simulink model "CAVE_MachE_Simulink_250904"  (R2024a)
settings: configuration reference "ConfigSetDesktopFixedStep" (kept outside this file)
PreLoadFcn:
  | VSS_BICYCLE=Simulink.Variant('Dual=0');
  | VSS_DUAL=Simulink.Variant('Dual=1');
  | Dual=1;
  | load('DriveCycle2.mat')
PostLoadFcn:
  | if any(exist('dsrtsu_mdlpostloadfcn', 'file') ~= 0), dsrtsu_mdlpostloadfcn('Execute', bdroot); end
InitFcn:
  | , if any(exist('rtifpga_mdlclblib', 'file') ~= 0), rtifpga_mdlclblib('Init', bdroot); end,
  | , if any(exist('dsmpb_private', 'file') ~= 0), dsmpb_private('dsmpb_mdlclblib', 'Init', bdroot); end,
  | load('DriveCycle2.mat')
model workspace (MAT data in the model file):
  Gas = 0.383333333333
undefined symbols (not defined in the file or in its folder): AccelCmd, ActTqLF_Nm_, ActTqLR_Nm_, ActTqRF_Nm_, ActTqRR_Nm_, BattChargeLimitMaxPwr, BattChargeLimitSocBpts, BattChargeLimitTbl, BattChrgCapcty, BattDischargeLimitSocBpts, BattDischargeLimitTbl, BattDischargeMaxPwr, BattNumCellsParallel, BattNumCellsSeries, BattOpenVoltCapBpts, BattOpenVoltTbl, BattResistSocBpts, BattResistTbl, BattResistTempBpts, BrakeMaxPrs, BrakeMaxTrq, ChassisDistCg2FrontAxle, ChassisDistCg2RearAxle, ChassisVehMass, CltchCmd, CoastDown, DecelCmd, DiffRatio, DiscIntNeverNeededParam, EnvGravCnst, EnvPrs, EnvTemp, FuelSpecificGrav, GearCmd, h, InitStates, lgSw, limitedMCT, MCT, MtrEffSpdBpts, MtrEffTbl, MtrEffTrqBpts, MtrPwrMax, MtrTrqMax, pMCT, RealSimPara, Ref_speed, Ref_time, SteeringCmd, SupvsryCtrlRegenBrkCutOffTbl, SupvsryCtrlRegenSpdBpts, TestScnrioCycleNum, US06, VEH
libraries: VSIGenLib x179, simulink x166, etargetslib x112, dsmpblib x58, vehdynlibtire x36, autolibshared x29, vehdynlibsuspension x21, vehdynlibtirecommon x21, autolibutils x15, CarMaker4SL x12, VsrLibWheel x12, autolibpowerinfoutils x9
(part 42 of 43)

== system CAVE_MachE_Simulink_250904/Vehicle Under Test3/Vehicle/Vehicle Dynamics/Vehicle 14DOF/Wheels and Tires/VDBS/Tires/MF Tires/omega1 ==
  In1 : Inport
  In2 : Inport  Port=2
  In3 : Inport  Port=3
  In4 : Inport  Port=4
  Abs{,1..3} (4 alike) : Abs  SaturateOnIntegerOverflow=off
  Constant : Constant  Value=0
  Rate Limiter{,1..3} (4 alike) : RateLimiter  RisingSlewLimit=5  FallingSlewLimit=-5  SampleTimeMode=inherited
  Switch{1..4} (4 alike) : Switch  Criteria=u2 > Threshold  Threshold=0.11  SaturateOnIntegerOverflow=off  InputSameDT=off
  Transfer Fcn{,1..3} (4 alike) : TransferFcn  Denominator=[0.1 1]
  Vector Concatenate : Concatenate  NumInputs=4
  Out1 : Outport  VectorParamsAs1DForOutWhenUnconnected=off
  wires:
  Vector Concatenate/1 -> Out1/1
  Abs2/1 -> Switch3/2
  Switch3/1 -> Vector Concatenate/3
  In4/1 -> Rate Limiter3/1
  Rate Limiter1/1 -> Transfer Fcn1/1
  Rate Limiter2/1 -> Transfer Fcn2/1
  In3/1 -> Rate Limiter2/1
  In1/1 -> Rate Limiter/1
  Switch4/1 -> Vector Concatenate/4
  Switch2/1 -> Vector Concatenate/2
  Rate Limiter/1 -> Transfer Fcn/1
  Transfer Fcn3/1 -> Abs3/1, Switch4/1
  Transfer Fcn1/1 -> Abs1/1, Switch2/1
  Constant/1 -> Switch4/3, Switch3/3, Switch2/3, Switch1/3
  Abs3/1 -> Switch4/2
  Switch1/1 -> Vector Concatenate/1
  Abs/1 -> Switch1/2
  Abs1/1 -> Switch2/2
  Transfer Fcn2/1 -> Abs2/1, Switch3/1
  Rate Limiter3/1 -> Transfer Fcn3/1
  In2/1 -> Rate Limiter1/1
  Transfer Fcn/1 -> Switch1/1, Abs/1

== system CAVE_MachE_Simulink_250904/Vehicle Under Test3/Vehicle/Vehicle Dynamics/Vehicle 14DOF/Wheels and Tires/VDBS/Tires/MF Tires/z ==
  In1 : Inport
  In2 : Inport  Port=2
  In3 : Inport  Port=3
  In4 : Inport  Port=4
  Bus Selector{,1..3} (4 alike) : BusSelector  OutputSignals=z
  Vector Concatenate : Concatenate  NumInputs=4
  Out1 : Outport  VectorParamsAs1DForOutWhenUnconnected=off
  wires:
  Bus Selector3/1 -> Vector Concatenate/4  "<z>"
  Bus Selector2/1 -> Vector Concatenate/3  "<z>"
  Bus Selector1/1 -> Vector Concatenate/2  "<z>"
  In4/1 -> Bus Selector3/1
  In3/1 -> Bus Selector2/1
  In2/1 -> Bus Selector1/1
  Bus Selector/1 -> Vector Concatenate/1  "<z>"
  In1/1 -> Bus Selector/1
  Vector Concatenate/1 -> Out1/1

== system CAVE_MachE_Simulink_250904/Vehicle Under Test3/Vehicle/Vehicle Dynamics/Vehicle 14DOF/Wheels and Tires/VDBS/Tires/MF Tires/zdot ==
  In1 : Inport
  In2 : Inport  Port=2
  In3 : Inport  Port=3
  In4 : Inport  Port=4
  Bus Selector{,1..3} (4 alike) : BusSelector  OutputSignals=zdot
  Vector Concatenate : Concatenate  NumInputs=4
  Out1 : Outport  VectorParamsAs1DForOutWhenUnconnected=off
  wires:
  Vector Concatenate/1 -> Out1/1
  In1/1 -> Bus Selector/1
  Bus Selector/1 -> Vector Concatenate/1  "<zdot>"
  In2/1 -> Bus Selector1/1
  In3/1 -> Bus Selector2/1
  In4/1 -> Bus Selector3/1
  Bus Selector1/1 -> Vector Concatenate/2  "<zdot>"
  Bus Selector2/1 -> Vector Concatenate/3  "<zdot>"
  Bus Selector3/1 -> Vector Concatenate/4  "<zdot>"

== system CAVE_MachE_Simulink_250904/Vehicle Under Test3/Vehicle/Vehicle Dynamics/Vehicle 14DOF/Wheels and Tires/VDBS/Veh2Tire/Wheel to Body Transform/Rotation Angles to Direction Cosine Matrix Retro: ZYX ==
  In1 : Inport
  Fcn : Fcn  Expr=u(5)*u(4)
  Fcn1 : Fcn  Expr=u(5)*u(1)
  Fcn2 : Fcn  Expr=-u(2)
  Fcn3 : Fcn  Expr=u(3)*u(2)*u(4)-u(6)*u(1)
  Fcn4 : Fcn  Expr=u(3)*u(2)*u(1)-u(6)*u(4)
  Fcn5 : Fcn  Expr=u(3)*u(5)
  Fcn6 : Fcn  Expr=u(6)*u(2)*u(4)-u(3)*u(1)
  Fcn7 : Fcn  Expr=u(6)*u(2)*u(1)-u(3)*u(4)
  Fcn8 : Fcn  Expr=u(6)*u(5)
  Mux : Mux  Inputs=2
  SinCos : Trigonometry  Operator=sincos
  Subsystem : Subsystem
  Out1 : Outport
  wires:
  Fcn1/1 -> Subsystem/2(In2)
  Mux/1 -> Fcn8/1, Fcn7/1, Fcn6/1, Fcn5/1, Fcn/1, Fcn1/1, Fcn2/1, Fcn3/1, Fcn4/1
  SinCos/2 -> Mux/2
  SinCos/1 -> Mux/1
  Fcn8/1 -> Subsystem/9(In9)
  Fcn7/1 -> Subsystem/8(In8)
  Fcn/1 -> Subsystem/1(In1)
  Fcn4/1 -> Subsystem/5(In5)
  In1/1 -> SinCos/1
  Fcn5/1 -> Subsystem/6(In6)
  Fcn2/1 -> Subsystem/3(In3)
  Fcn3/1 -> Subsystem/4(In4)
  Fcn6/1 -> Subsystem/7(In7)
  Subsystem/1(Out1) -> Out1/1

== system CAVE_MachE_Simulink_250904/Vehicle Under Test4/Vehicle/Vehicle Dynamics/Vehicle 14DOF/Wheels and Tires/VDBS/Tire2Veh/Wheel to Body Transform/Rotation Angles to Direction Cosine Matrix Retro: ZYX ==
  In1 : Inport
  Fcn : Fcn  Expr=u(5)*u(4)
  Fcn1 : Fcn  Expr=u(5)*u(1)
  Fcn2 : Fcn  Expr=-u(2)
  Fcn3 : Fcn  Expr=u(3)*u(2)*u(4)-u(6)*u(1)
  Fcn4 : Fcn  Expr=u(3)*u(2)*u(1)-u(6)*u(4)
  Fcn5 : Fcn  Expr=u(3)*u(5)
  Fcn6 : Fcn  Expr=u(6)*u(2)*u(4)-u(3)*u(1)
  Fcn7 : Fcn  Expr=u(6)*u(2)*u(1)-u(3)*u(4)
  Fcn8 : Fcn  Expr=u(6)*u(5)
  Mux : Mux  Inputs=2
  SinCos : Trigonometry  Operator=sincos
  Subsystem : Subsystem
  Out1 : Outport
  wires:
  Subsystem/1(Out1) -> Out1/1
  Fcn6/1 -> Subsystem/7(In7)
  Fcn3/1 -> Subsystem/4(In4)
  Fcn2/1 -> Subsystem/3(In3)
  Fcn5/1 -> Subsystem/6(In6)
  In1/1 -> SinCos/1
  Fcn4/1 -> Subsystem/5(In5)
  Fcn/1 -> Subsystem/1(In1)
  Fcn7/1 -> Subsystem/8(In8)
  Fcn8/1 -> Subsystem/9(In9)
  SinCos/1 -> Mux/1
  SinCos/2 -> Mux/2
  Mux/1 -> Fcn4/1, Fcn3/1, Fcn2/1, Fcn1/1, Fcn/1, Fcn5/1, Fcn6/1, Fcn7/1, Fcn8/1
  Fcn1/1 -> Subsystem/2(In2)

== system CAVE_MachE_Simulink_250904/Vehicle Under Test4/Vehicle/Vehicle Dynamics/Vehicle 14DOF/Wheels and Tires/VDBS/Tires/Fiala Tires/Fx ==
  In1 : Inport
  In2 : Inport  Port=2
  In3 : Inport  Port=3
  In4 : Inport  Port=4
  Bus Selector{,1..3} (4 alike) : BusSelector  OutputSignals=Fx
  Vector Concatenate : Concatenate  NumInputs=4
  Out1 : Outport  VectorParamsAs1DForOutWhenUnconnected=off
  wires:
  Vector Concatenate/1 -> Out1/1
  In1/1 -> Bus Selector/1
  Bus Selector/1 -> Vector Concatenate/1  "<Fx>"
  In2/1 -> Bus Selector1/1
  In3/1 -> Bus Selector2/1
  In4/1 -> Bus Selector3/1
  Bus Selector1/1 -> Vector Concatenate/2  "<Fx>"
  Bus Selector2/1 -> Vector Concatenate/3  "<Fx>"
  Bus Selector3/1 -> Vector Concatenate/4  "<Fx>"

== system CAVE_MachE_Simulink_250904/Vehicle Under Test4/Vehicle/Vehicle Dynamics/Vehicle 14DOF/Wheels and Tires/VDBS/Tires/Fiala Tires/Fy ==
  In1 : Inport
  In2 : Inport  Port=2
  In3 : Inport  Port=3
  In4 : Inport  Port=4
  Bus Selector{,1..3} (4 alike) : BusSelector  OutputSignals=Fy
  Vector Concatenate : Concatenate  NumInputs=4
  Out1 : Outport  VectorParamsAs1DForOutWhenUnconnected=off
  wires:
  Bus Selector3/1 -> Vector Concatenate/4  "<Fy>"
  Bus Selector2/1 -> Vector Concatenate/3  "<Fy>"
  Bus Selector1/1 -> Vector Concatenate/2  "<Fy>"
  In4/1 -> Bus Selector3/1
  In3/1 -> Bus Selector2/1
  In2/1 -> Bus Selector1/1
  Bus Selector/1 -> Vector Concatenate/1  "<Fy>"
  In1/1 -> Bus Selector/1
  Vector Concatenate/1 -> Out1/1

== system CAVE_MachE_Simulink_250904/Vehicle Under Test4/Vehicle/Vehicle Dynamics/Vehicle 14DOF/Wheels and Tires/VDBS/Tires/Fiala Tires/Fz ==
  In1 : Inport
  In2 : Inport  Port=2
  In3 : Inport  Port=3
  In4 : Inport  Port=4
  Bus Selector{,1..3} (4 alike) : BusSelector  OutputSignals=Fz
  Vector Concatenate : Concatenate  NumInputs=4
  Out1 : Outport  VectorParamsAs1DForOutWhenUnconnected=off
  wires:
  Bus Selector3/1 -> Vector Concatenate/4  "<Fz>"
  Bus Selector2/1 -> Vector Concatenate/3  "<Fz>"
  Bus Selector1/1 -> Vector Concatenate/2  "<Fz>"
  In4/1 -> Bus Selector3/1
  In3/1 -> Bus Selector2/1
  In2/1 -> Bus Selector1/1
  Bus Selector/1 -> Vector Concatenate/1  "<Fz>"
  In1/1 -> Bus Selector/1
  Vector Concatenate/1 -> Out1/1

== system CAVE_MachE_Simulink_250904/Vehicle Under Test4/Vehicle/Vehicle Dynamics/Vehicle 14DOF/Wheels and Tires/VDBS/Tires/Fiala Tires/Mx ==
  In1 : Inport
  In2 : Inport  Port=2
  In3 : Inport  Port=3
  In4 : Inport  Port=4
  Bus Selector{,1..3} (4 alike) : BusSelector  OutputSignals=Mx
  Vector Concatenate : Concatenate  NumInputs=4
  Out1 : Outport  VectorParamsAs1DForOutWhenUnconnected=off
  wires:
  Bus Selector3/1 -> Vector Concatenate/4  "<Mx>"
  Bus Selector2/1 -> Vector Concatenate/3  "<Mx>"
  Bus Selector1/1 -> Vector Concatenate/2  "<Mx>"
  In4/1 -> Bus Selector3/1
  In3/1 -> Bus Selector2/1
  In2/1 -> Bus Selector1/1
  Bus Selector/1 -> Vector Concatenate/1  "<Mx>"
  In1/1 -> Bus Selector/1
  Vector Concatenate/1 -> Out1/1

== system CAVE_MachE_Simulink_250904/Vehicle Under Test4/Vehicle/Vehicle Dynamics/Vehicle 14DOF/Wheels and Tires/VDBS/Tires/Fiala Tires/My ==
  In1 : Inport
  In2 : Inport  Port=2
  In3 : Inport  Port=3
  In4 : Inport  Port=4
  Bus Selector{,1..3} (4 alike) : BusSelector  OutputSignals=My
  Vector Concatenate : Concatenate  NumInputs=4
  Out1 : Outport  VectorParamsAs1DForOutWhenUnconnected=off
  wires:
  Vector Concatenate/1 -> Out1/1
  In1/1 -> Bus Selector/1
  Bus Selector/1 -> Vector Concatenate/1  "<My>"
  In2/1 -> Bus Selector1/1
  In3/1 -> Bus Selector2/1
  In4/1 -> Bus Selector3/1
  Bus Selector1/1 -> Vector Concatenate/2  "<My>"
  Bus Selector2/1 -> Vector Concatenate/3  "<My>"
  Bus Selector3/1 -> Vector Concatenate/4  "<My>"

== system CAVE_MachE_Simulink_250904/Vehicle Under Test4/Vehicle/Vehicle Dynamics/Vehicle 14DOF/Wheels and Tires/VDBS/Tires/Fiala Tires/Mz ==
  In1 : Inport
  In2 : Inport  Port=2
  In3 : Inport  Port=3
  In4 : Inport  Port=4
  Bus Selector{,1..3} (4 alike) : BusSelector  OutputSignals=Mz
  Vector Concatenate : Concatenate  NumInputs=4
  Out1 : Outport  VectorParamsAs1DForOutWhenUnconnected=off
  wires:
  Vector Concatenate/1 -> Out1/1
  In1/1 -> Bus Selector/1
  Bus Selector/1 -> Vector Concatenate/1  "<Mz>"
  In2/1 -> Bus Selector1/1
  In3/1 -> Bus Selector2/1
  In4/1 -> Bus Selector3/1
  Bus Selector1/1 -> Vector Concatenate/2  "<Mz>"
  Bus Selector2/1 -> Vector Concatenate/3  "<Mz>"
  Bus Selector3/1 -> Vector Concatenate/4  "<Mz>"

== system CAVE_MachE_Simulink_250904/Vehicle Under Test4/Vehicle/Vehicle Dynamics/Vehicle 14DOF/Wheels and Tires/VDBS/Tires/Fiala Tires/Re ==
  In1 : Inport
  In2 : Inport  Port=2
  In3 : Inport  Port=3
  In4 : Inport  Port=4
  Bus Selector{,1..3} (4 alike) : BusSelector  OutputSignals=Re
  Vector Concatenate : Concatenate  NumInputs=4
  Out1 : Outport  VectorParamsAs1DForOutWhenUnconnected=off
  wires:
  Bus Selector3/1 -> Vector Concatenate/4  "<Re>"
  Bus Selector2/1 -> Vector Concatenate/3  "<Re>"
  Bus Selector1/1 -> Vector Concatenate/2  "<Re>"
  In4/1 -> Bus Selector3/1
  In3/1 -> Bus Selector2/1
  In2/1 -> Bus Selector1/1
  Bus Selector/1 -> Vector Concatenate/1  "<Re>"
  In1/1 -> Bus Selector/1
  Vector Concatenate/1 -> Out1/1

== system CAVE_MachE_Simulink_250904/Vehicle Under Test4/Vehicle/Vehicle Dynamics/Vehicle 14DOF/Wheels and Tires/VDBS/Tires/Fiala Tires/alpha ==
  In1 : Inport
  In2 : Inport  Port=2
  In3 : Inport  Port=3
  In4 : Inport  Port=4
  Bus Selector{,1..3} (4 alike) : BusSelector  OutputSignals=Alpha
  Vector Concatenate : Concatenate  NumInputs=4
  Out1 : Outport  VectorParamsAs1DForOutWhenUnconnected=off
  wires:
  Bus Selector3/1 -> Vector Concatenate/4  "<Alpha>"
  Bus Selector2/1 -> Vector Concatenate/3  "<Alpha>"
  Bus Selector1/1 -> Vector Concatenate/2  "<Alpha>"
  In4/1 -> Bus Selector3/1
  In3/1 -> Bus Selector2/1
  In2/1 -> Bus Selector1/1
  Bus Selector/1 -> Vector Concatenate/1  "<Alpha>"
  In1/1 -> Bus Selector/1
  Vector Concatenate/1 -> Out1/1

== system CAVE_MachE_Simulink_250904/Vehicle Under Test4/Vehicle/Vehicle Dynamics/Vehicle 14DOF/Wheels and Tires/VDBS/Tires/Fiala Tires/kappa ==
  In1 : Inport
  In2 : Inport  Port=2
  In3 : Inport  Port=3
  In4 : Inport  Port=4
  Bus Selector{,1..3} (4 alike) : BusSelector  OutputSignals=Kappa
  Vector Concatenate : Concatenate  NumInputs=4
  Out1 : Outport  VectorParamsAs1DForOutWhenUnconnected=off
  wires:
  Vector Concatenate/1 -> Out1/1
  In1/1 -> Bus Selector/1
  Bus Selector/1 -> Vector Concatenate/1  "<Kappa>"
  In2/1 -> Bus Selector1/1
  In3/1 -> Bus Selector2/1
  In4/1 -> Bus Selector3/1
  Bus Selector1/1 -> Vector Concatenate/2  "<Kappa>"
  Bus Selector2/1 -> Vector Concatenate/3  "<Kappa>"
  Bus Selector3/1 -> Vector Concatenate/4  "<Kappa>"

== system CAVE_MachE_Simulink_250904/Vehicle Under Test4/Vehicle/Vehicle Dynamics/Vehicle 14DOF/Wheels and Tires/VDBS/Tires/Fiala Tires/omega ==
  In1 : Inport
  In2 : Inport  Port=2
  In3 : Inport  Port=3
  In4 : Inport  Port=4
  Bus Selector{,1..3} (4 alike) : BusSelector  OutputSignals=Omega
  Vector Concatenate : Concatenate  NumInputs=4
  Out1 : Outport  VectorParamsAs1DForOutWhenUnconnected=off
  wires:
  Vector Concatenate/1 -> Out1/1
  Bus Selector3/1 -> Vector Concatenate/4  "<Omega>"
  Bus Selector2/1 -> Vector Concatenate/3  "<Omega>"
  Bus Selector1/1 -> Vector Concatenate/2  "<Omega>"
  In4/1 -> Bus Selector3/1
  In3/1 -> Bus Selector2/1
  In2/1 -> Bus Selector1/1
  Bus Selector/1 -> Vector Concatenate/1  "<Omega>"
  In1/1 -> Bus Selector/1

== system CAVE_MachE_Simulink_250904/Vehicle Under Test4/Vehicle/Vehicle Dynamics/Vehicle 14DOF/Wheels and Tires/VDBS/Tires/Fiala Tires/z ==
  In1 : Inport
  In2 : Inport  Port=2
  In3 : Inport  Port=3
  In4 : Inport  Port=4
  Bus Selector{,1..3} (4 alike) : BusSelector  OutputSignals=z
  Vector Concatenate : Concatenate  NumInputs=4
  Out1 : Outport  VectorParamsAs1DForOutWhenUnconnected=off
  wires:
  Vector Concatenate/1 -> Out1/1
  In1/1 -> Bus Selector/1
  Bus Selector/1 -> Vector Concatenate/1  "<z>"
  In2/1 -> Bus Selector1/1
  In3/1 -> Bus Selector2/1
  In4/1 -> Bus Selector3/1
  Bus Selector1/1 -> Vector Concatenate/2  "<z>"
  Bus Selector2/1 -> Vector Concatenate/3  "<z>"
  Bus Selector3/1 -> Vector Concatenate/4  "<z>"

== system CAVE_MachE_Simulink_250904/Vehicle Under Test4/Vehicle/Vehicle Dynamics/Vehicle 14DOF/Wheels and Tires/VDBS/Tires/Fiala Tires/zdot ==
  In1 : Inport
  In2 : Inport  Port=2
  In3 : Inport  Port=3
  In4 : Inport  Port=4
  Bus Selector{,1..3} (4 alike) : BusSelector  OutputSignals=zdot
  Vector Concatenate : Concatenate  NumInputs=4
  Out1 : Outport  VectorParamsAs1DForOutWhenUnconnected=off
  wires:
  Bus Selector3/1 -> Vector Concatenate/4  "<zdot>"
  Bus Selector2/1 -> Vector Concatenate/3  "<zdot>"
  Bus Selector1/1 -> Vector Concatenate/2  "<zdot>"
  In4/1 -> Bus Selector3/1
  In3/1 -> Bus Selector2/1
  In2/1 -> Bus Selector1/1
  Bus Selector/1 -> Vector Concatenate/1  "<zdot>"
  In1/1 -> Bus Selector/1
  Vector Concatenate/1 -> Out1/1

== system CAVE_MachE_Simulink_250904/Vehicle Under Test4/Vehicle/Vehicle Dynamics/Vehicle 14DOF/Wheels and Tires/VDBS/Tires/MF Tires/Fx ==
  In1 : Inport
  In2 : Inport  Port=2
  In3 : Inport  Port=3
  In4 : Inport  Port=4
  Bus Selector{,1..3} (4 alike) : BusSelector  OutputSignals=Fx
  Vector Concatenate : Concatenate  NumInputs=4
  Out1 : Outport  VectorParamsAs1DForOutWhenUnconnected=off
  wires:
  Vector Concatenate/1 -> Out1/1
  In1/1 -> Bus Selector/1
  Bus Selector/1 -> Vector Concatenate/1  "<Fx>"
  In2/1 -> Bus Selector1/1
  In3/1 -> Bus Selector2/1
  In4/1 -> Bus Selector3/1
  Bus Selector1/1 -> Vector Concatenate/2  "<Fx>"
  Bus Selector2/1 -> Vector Concatenate/3  "<Fx>"
  Bus Selector3/1 -> Vector Concatenate/4  "<Fx>"

== system CAVE_MachE_Simulink_250904/Vehicle Under Test4/Vehicle/Vehicle Dynamics/Vehicle 14DOF/Wheels and Tires/VDBS/Tires/MF Tires/Fy ==
  In1 : Inport
  In2 : Inport  Port=2
  In3 : Inport  Port=3
  In4 : Inport  Port=4
  Bus Selector{,1..3} (4 alike) : BusSelector  OutputSignals=Fy
  Vector Concatenate : Concatenate  NumInputs=4
  Out1 : Outport  VectorParamsAs1DForOutWhenUnconnected=off
  wires:
  Bus Selector3/1 -> Vector Concatenate/4  "<Fy>"
  Bus Selector2/1 -> Vector Concatenate/3  "<Fy>"
  Bus Selector1/1 -> Vector Concatenate/2  "<Fy>"
  In4/1 -> Bus Selector3/1
  In3/1 -> Bus Selector2/1
  In2/1 -> Bus Selector1/1
  Bus Selector/1 -> Vector Concatenate/1  "<Fy>"
  In1/1 -> Bus Selector/1
  Vector Concatenate/1 -> Out1/1

== system CAVE_MachE_Simulink_250904/Vehicle Under Test4/Vehicle/Vehicle Dynamics/Vehicle 14DOF/Wheels and Tires/VDBS/Tires/MF Tires/Fz ==
  In1 : Inport
  In2 : Inport  Port=2
  In3 : Inport  Port=3
  In4 : Inport  Port=4
  Bus Selector{,1..3} (4 alike) : BusSelector  OutputSignals=Fz
  Vector Concatenate : Concatenate  NumInputs=4
  Out1 : Outport  VectorParamsAs1DForOutWhenUnconnected=off
  wires:
  Bus Selector3/1 -> Vector Concatenate/4  "<Fz>"
  Bus Selector2/1 -> Vector Concatenate/3  "<Fz>"
  Bus Selector1/1 -> Vector Concatenate/2  "<Fz>"
  In4/1 -> Bus Selector3/1
  In3/1 -> Bus Selector2/1
  In2/1 -> Bus Selector1/1
  Bus Selector/1 -> Vector Concatenate/1  "<Fz>"
  In1/1 -> Bus Selector/1
  Vector Concatenate/1 -> Out1/1

== system CAVE_MachE_Simulink_250904/Vehicle Under Test4/Vehicle/Vehicle Dynamics/Vehicle 14DOF/Wheels and Tires/VDBS/Tires/MF Tires/Mx ==
  In1 : Inport
  In2 : Inport  Port=2
  In3 : Inport  Port=3
  In4 : Inport  Port=4
  Bus Selector{,1..3} (4 alike) : BusSelector  Commented=on  OutputSignals=Mx
  Vector Concatenate : Concatenate  NumInputs=4
  Out1 : Outport  VectorParamsAs1DForOutWhenUnconnected=off
  wires:
  In4/1 -> Vector Concatenate/4
  In3/1 -> Vector Concatenate/3
  In2/1 -> Vector Concatenate/2
  In1/1 -> Vector Concatenate/1
  Bus Selector1/1 -> ?  "<Mx>"
  ? -> Bus Selector3/1
  ? -> Bus Selector/1
  Bus Selector2/1 -> ?  "<Mx>"
  Bus Selector/1 -> ?  "<Mx>"
  Bus Selector3/1 -> ?  "<Mx>"
  ? -> Bus Selector1/1
  ? -> Bus Selector2/1
  Vector Concatenate/1 -> Out1/1

== system CAVE_MachE_Simulink_250904/Vehicle Under Test4/Vehicle/Vehicle Dynamics/Vehicle 14DOF/Wheels and Tires/VDBS/Tires/MF Tires/My ==
  In1 : Inport
  In2 : Inport  Port=2
  In3 : Inport  Port=3
  In4 : Inport  Port=4
  Bus Selector{,1..3} (4 alike) : BusSelector  OutputSignals=My
  Vector Concatenate : Concatenate  NumInputs=4
  Out1 : Outport  VectorParamsAs1DForOutWhenUnconnected=off
  wires:
  Vector Concatenate/1 -> Out1/1
  In1/1 -> Bus Selector/1
  Bus Selector/1 -> Vector Concatenate/1  "<My>"
  In2/1 -> Bus Selector1/1
  In3/1 -> Bus Selector2/1
  In4/1 -> Bus Selector3/1
  Bus Selector1/1 -> Vector Concatenate/2  "<My>"
  Bus Selector2/1 -> Vector Concatenate/3  "<My>"
  Bus Selector3/1 -> Vector Concatenate/4  "<My>"

== system CAVE_MachE_Simulink_250904/Vehicle Under Test4/Vehicle/Vehicle Dynamics/Vehicle 14DOF/Wheels and Tires/VDBS/Tires/MF Tires/Mz ==
  In1 : Inport
  In2 : Inport  Port=2
  In3 : Inport  Port=3
  In4 : Inport  Port=4
  Bus Selector{,1..3} (4 alike) : BusSelector  Commented=on  OutputSignals=Mz
  Vector Concatenate : Concatenate  NumInputs=4
  Out1 : Outport  VectorParamsAs1DForOutWhenUnconnected=off
  wires:
  In4/1 -> Vector Concatenate/4
  In3/1 -> Vector Concatenate/3
  In2/1 -> Vector Concatenate/2
  In1/1 -> Vector Concatenate/1
  Bus Selector1/1 -> ?  "<Mz>"
  Bus Selector/1 -> ?  "<Mz>"
  ? -> Bus Selector3/1
  Bus Selector3/1 -> ?  "<Mz>"
  ? -> Bus Selector2/1
  ? -> Bus Selector1/1
  Bus Selector2/1 -> ?  "<Mz>"
  ? -> Bus Selector/1
  Vector Concatenate/1 -> Out1/1

== system CAVE_MachE_Simulink_250904/Vehicle Under Test4/Vehicle/Vehicle Dynamics/Vehicle 14DOF/Wheels and Tires/VDBS/Tires/MF Tires/Re ==
  In1 : Inport
  In2 : Inport  Port=2
  In3 : Inport  Port=3
  In4 : Inport  Port=4
  Bus Selector{,1..3} (4 alike) : BusSelector  OutputSignals=Re
  Vector Concatenate : Concatenate  NumInputs=4
  Out1 : Outport  VectorParamsAs1DForOutWhenUnconnected=off
  wires:
  Bus Selector3/1 -> Vector Concatenate/4  "<Re>"
  Bus Selector2/1 -> Vector Concatenate/3  "<Re>"
  Bus Selector1/1 -> Vector Concatenate/2  "<Re>"
  In4/1 -> Bus Selector3/1
  In3/1 -> Bus Selector2/1
  In2/1 -> Bus Selector1/1
  Bus Selector/1 -> Vector Concatenate/1  "<Re>"
  In1/1 -> Bus Selector/1
  Vector Concatenate/1 -> Out1/1

== system CAVE_MachE_Simulink_250904/Vehicle Under Test4/Vehicle/Vehicle Dynamics/Vehicle 14DOF/Wheels and Tires/VDBS/Tires/MF Tires/alpha ==
  In1 : Inport
  In2 : Inport  Port=2
  In3 : Inport  Port=3
  In4 : Inport  Port=4
  Bus Selector{,1..3} (4 alike) : BusSelector  OutputSignals=Alpha
  Vector Concatenate : Concatenate  NumInputs=4
  Out1 : Outport  VectorParamsAs1DForOutWhenUnconnected=off
  wires:
  Bus Selector3/1 -> Vector Concatenate/4  "<Alpha>"
  Bus Selector2/1 -> Vector Concatenate/3  "<Alpha>"
  Bus Selector1/1 -> Vector Concatenate/2  "<Alpha>"
  In4/1 -> Bus Selector3/1
  In3/1 -> Bus Selector2/1
  In2/1 -> Bus Selector1/1
  Bus Selector/1 -> Vector Concatenate/1  "<Alpha>"
  In1/1 -> Bus Selector/1
  Vector Concatenate/1 -> Out1/1

== system CAVE_MachE_Simulink_250904/Vehicle Under Test4/Vehicle/Vehicle Dynamics/Vehicle 14DOF/Wheels and Tires/VDBS/Tires/MF Tires/kappa ==
  In1 : Inport
  In2 : Inport  Port=2
  In3 : Inport  Port=3
  In4 : Inport  Port=4
  Bus Selector{,1..3} (4 alike) : BusSelector  OutputSignals=Kappa
  Vector Concatenate : Concatenate  NumInputs=4
  Out1 : Outport  VectorParamsAs1DForOutWhenUnconnected=off
  wires:
  Vector Concatenate/1 -> Out1/1
  In1/1 -> Bus Selector/1
  Bus Selector/1 -> Vector Concatenate/1  "<Kappa>"
  In2/1 -> Bus Selector1/1
  In3/1 -> Bus Selector2/1
  In4/1 -> Bus Selector3/1
  Bus Selector1/1 -> Vector Concatenate/2  "<Kappa>"
  Bus Selector2/1 -> Vector Concatenate/3  "<Kappa>"
  Bus Selector3/1 -> Vector Concatenate/4  "<Kappa>"

== system CAVE_MachE_Simulink_250904/Vehicle Under Test4/Vehicle/Vehicle Dynamics/Vehicle 14DOF/Wheels and Tires/VDBS/Tires/MF Tires/omega ==
  In1 : Inport
  In2 : Inport  Port=2
  In3 : Inport  Port=3
  In4 : Inport  Port=4
  Abs{,1..3} (4 alike) : Abs  SaturateOnIntegerOverflow=off
  Bus Selector{,1..3} (4 alike) : BusSelector  OutputSignals=Omega
  Constant : Constant  Value=0
  Rate Limiter{4..7} (4 alike) : RateLimiter  Commented=on  RisingSlewLimit=3  FallingSlewLimit=-3  SampleTimeMode=inherited
  Scope : Scope  NumInputPorts=2
  Scope1 : Scope  NumInputPorts=4
  Switch{1..4} (4 alike) : Switch  Criteria=u2 > Threshold  Threshold=0.11  SaturateOnIntegerOverflow=off  InputSameDT=off
  Transfer Fcn{,1..3} (4 alike) : TransferFcn  Denominator=[0.1 1]
  Vector Concatenate : Concatenate  NumInputs=4
  Out1 : Outport  VectorParamsAs1DForOutWhenUnconnected=off
  wires:
  Transfer Fcn/1 -> Abs/1, Switch1/1
  Bus Selector1/1 -> Transfer Fcn1/1, Scope1/2  "<Omega>"
  Transfer Fcn2/1 -> Switch3/1, Abs2/1
  Abs1/1 -> Switch2/2
  Abs/1 -> Switch1/2
  Switch1/1 -> Scope/2, Vector Concatenate/1
  Abs3/1 -> Switch4/2
  Constant/1 -> Switch1/3, Switch2/3, Switch3/3, Switch4/3
  Transfer Fcn1/1 -> Switch2/1, Abs1/1
  Transfer Fcn3/1 -> Switch4/1, Abs3/1
  Switch2/1 -> Vector Concatenate/2
  Switch4/1 -> Vector Concatenate/4
  Bus Selector/1 -> Scope/1, Scope1/1, Transfer Fcn/1  "<Omega>"
  Bus Selector2/1 -> Scope1/3, Transfer Fcn2/1  "<Omega>"
  Bus Selector3/1 -> Scope1/4, Transfer Fcn3/1  "<Omega>"
  Switch3/1 -> Vector Concatenate/3
  Abs2/1 -> Switch3/2
  Vector Concatenate/1 -> Out1/1
  In4/1 -> Bus Selector3/1
  In3/1 -> Bus Selector2/1
  In2/1 -> Bus Selector1/1
  In1/1 -> Bus Selector/1

== system CAVE_MachE_Simulink_250904/Vehicle Under Test4/Vehicle/Vehicle Dynamics/Vehicle 14DOF/Wheels and Tires/VDBS/Tires/MF Tires/omega1 ==
  In1 : Inport
  In2 : Inport  Port=2
  In3 : Inport  Port=3
  In4 : Inport  Port=4
  Abs{,1..3} (4 alike) : Abs  SaturateOnIntegerOverflow=off
  Constant : Constant  Value=0
  Rate Limiter{,1..3} (4 alike) : RateLimiter  RisingSlewLimit=5  FallingSlewLimit=-5  SampleTimeMode=inherited
  Switch{1..4} (4 alike) : Switch  Criteria=u2 > Threshold  Threshold=0.11  SaturateOnIntegerOverflow=off  InputSameDT=off
  Transfer Fcn{,1..3} (4 alike) : TransferFcn  Denominator=[0.1 1]
  Vector Concatenate : Concatenate  NumInputs=4
  Out1 : Outport  VectorParamsAs1DForOutWhenUnconnected=off
  wires:
  Transfer Fcn/1 -> Abs/1, Switch1/1
  In2/1 -> Rate Limiter1/1
  Rate Limiter3/1 -> Transfer Fcn3/1
  Transfer Fcn2/1 -> Switch3/1, Abs2/1
  Abs1/1 -> Switch2/2
  Abs/1 -> Switch1/2
  Switch1/1 -> Vector Concatenate/1
  Abs3/1 -> Switch4/2
  Constant/1 -> Switch1/3, Switch2/3, Switch3/3, Switch4/3
  Transfer Fcn1/1 -> Switch2/1, Abs1/1
  Transfer Fcn3/1 -> Switch4/1, Abs3/1
  Rate Limiter/1 -> Transfer Fcn/1
  Switch2/1 -> Vector Concatenate/2
  Switch4/1 -> Vector Concatenate/4
  In1/1 -> Rate Limiter/1
  In3/1 -> Rate Limiter2/1
  Rate Limiter2/1 -> Transfer Fcn2/1
  Rate Limiter1/1 -> Transfer Fcn1/1
  In4/1 -> Rate Limiter3/1
  Switch3/1 -> Vector Concatenate/3
  Abs2/1 -> Switch3/2
  Vector Concatenate/1 -> Out1/1

== system CAVE_MachE_Simulink_250904/Vehicle Under Test4/Vehicle/Vehicle Dynamics/Vehicle 14DOF/Wheels and Tires/VDBS/Tires/MF Tires/z ==
  In1 : Inport
  In2 : Inport  Port=2
  In3 : Inport  Port=3
  In4 : Inport  Port=4
  Bus Selector{,1..3} (4 alike) : BusSelector  OutputSignals=z
  Vector Concatenate : Concatenate  NumInputs=4
  Out1 : Outport  VectorParamsAs1DForOutWhenUnconnected=off
  wires:
  Vector Concatenate/1 -> Out1/1
  In1/1 -> Bus Selector/1
  Bus Selector/1 -> Vector Concatenate/1  "<z>"
  In2/1 -> Bus Selector1/1
  In3/1 -> Bus Selector2/1
  In4/1 -> Bus Selector3/1
  Bus Selector1/1 -> Vector Concatenate/2  "<z>"
  Bus Selector2/1 -> Vector Concatenate/3  "<z>"
  Bus Selector3/1 -> Vector Concatenate/4  "<z>"

== system CAVE_MachE_Simulink_250904/Vehicle Under Test4/Vehicle/Vehicle Dynamics/Vehicle 14DOF/Wheels and Tires/VDBS/Tires/MF Tires/zdot ==
  In1 : Inport
  In2 : Inport  Port=2
  In3 : Inport  Port=3
  In4 : Inport  Port=4
  Bus Selector{,1..3} (4 alike) : BusSelector  OutputSignals=zdot
  Vector Concatenate : Concatenate  NumInputs=4
  Out1 : Outport  VectorParamsAs1DForOutWhenUnconnected=off
  wires:
  Bus Selector3/1 -> Vector Concatenate/4  "<zdot>"
  Bus Selector2/1 -> Vector Concatenate/3  "<zdot>"
  Bus Selector1/1 -> Vector Concatenate/2  "<zdot>"
  In4/1 -> Bus Selector3/1
  In3/1 -> Bus Selector2/1
  In2/1 -> Bus Selector1/1
  Bus Selector/1 -> Vector Concatenate/1  "<zdot>"
  In1/1 -> Bus Selector/1
  Vector Concatenate/1 -> Out1/1

== system CAVE_MachE_Simulink_250904/Vehicle Under Test4/Vehicle/Vehicle Dynamics/Vehicle 14DOF/Wheels and Tires/VDBS/Veh2Tire/Wheel to Body Transform/Rotation Angles to Direction Cosine Matrix Retro: ZYX ==
  In1 : Inport
  Fcn : Fcn  Expr=u(5)*u(4)
  Fcn1 : Fcn  Expr=u(5)*u(1)
  Fcn2 : Fcn  Expr=-u(2)
  Fcn3 : Fcn  Expr=u(3)*u(2)*u(4)-u(6)*u(1)
  Fcn4 : Fcn  Expr=u(3)*u(2)*u(1)-u(6)*u(4)
  Fcn5 : Fcn  Expr=u(3)*u(5)
  Fcn6 : Fcn  Expr=u(6)*u(2)*u(4)-u(3)*u(1)
  Fcn7 : Fcn  Expr=u(6)*u(2)*u(1)-u(3)*u(4)
  Fcn8 : Fcn  Expr=u(6)*u(5)
  Mux : Mux  Inputs=2
  SinCos : Trigonometry  Operator=sincos
  Subsystem : Subsystem
  Out1 : Outport
  wires:
  Subsystem/1(Out1) -> Out1/1
  Fcn6/1 -> Subsystem/7(In7)
  Fcn3/1 -> Subsystem/4(In4)
  Fcn2/1 -> Subsystem/3(In3)
  Fcn5/1 -> Subsystem/6(In6)
  In1/1 -> SinCos/1
  Fcn4/1 -> Subsystem/5(In5)
  Fcn/1 -> Subsystem/1(In1)
  Fcn7/1 -> Subsystem/8(In8)
  Fcn8/1 -> Subsystem/9(In9)
  SinCos/1 -> Mux/1
  SinCos/2 -> Mux/2
  Mux/1 -> Fcn4/1, Fcn3/1, Fcn2/1, Fcn1/1, Fcn/1, Fcn5/1, Fcn6/1, Fcn7/1, Fcn8/1
  Fcn1/1 -> Subsystem/2(In2)

== system CAVE_MachE_Simulink_250904/Vehicle Under Test1/Vehicle/Vehicle Dynamics/Vehicle 14DOF/Wheels and Tires/VDBS/Tire2Veh/Wheel to Body Transform/Rotation Angles to Direction Cosine Matrix Retro: ZYX/Subsystem ==
  In1 : Inport
  In2 : Inport  Port=2
  In3 : Inport  Port=3
  In4 : Inport  Port=4
  In5 : Inport  Port=5
  In6 : Inport  Port=6
  In7 : Inport  Port=7
  In8 : Inport  Port=8
  In9 : Inport  Port=9
  Reshape : Reshape  OutputDimensionality=Customize  OutputDimensions=[3, 3]
  Vector Concatenate : Concatenate  NumInputs=9
  Out1 : Outport
  wires:
  In9/1 -> Vector Concatenate/9
  In6/1 -> Vector Concatenate/8
  In3/1 -> Vector Concatenate/7
  In8/1 -> Vector Concatenate/6
  In5/1 -> Vector Concatenate/5
  In2/1 -> Vector Concatenate/4
  In7/1 -> Vector Concatenate/3
  In4/1 -> Vector Concatenate/2
  In1/1 -> Vector Concatenate/1
  Vector Concatenate/1 -> Reshape/1
  Reshape/1 -> Out1/1

== system CAVE_MachE_Simulink_250904/Vehicle Under Test1/Vehicle/Vehicle Dynamics/Vehicle 14DOF/Wheels and Tires/VDBS/Veh2Tire/Wheel to Body Transform/Rotation Angles to Direction Cosine Matrix Retro: ZYX/Subsystem ==
  In1 : Inport
  In2 : Inport  Port=2
  In3 : Inport  Port=3
  In4 : Inport  Port=4
  In5 : Inport  Port=5
  In6 : Inport  Port=6
  In7 : Inport  Port=7
  In8 : Inport  Port=8
  In9 : Inport  Port=9
  Reshape : Reshape  OutputDimensionality=Customize  OutputDimensions=[3, 3]
  Vector Concatenate : Concatenate  NumInputs=9
  Out1 : Outport
  wires:
  In9/1 -> Vector Concatenate/9
  In6/1 -> Vector Concatenate/8
  In3/1 -> Vector Concatenate/7
  In8/1 -> Vector Concatenate/6
  In5/1 -> Vector Concatenate/5
  In2/1 -> Vector Concatenate/4
  In7/1 -> Vector Concatenate/3
  In4/1 -> Vector Concatenate/2
  In1/1 -> Vector Concatenate/1
  Vector Concatenate/1 -> Reshape/1
  Reshape/1 -> Out1/1

== system CAVE_MachE_Simulink_250904/Vehicle Under Test3/Vehicle/Vehicle Dynamics/Vehicle 14DOF/Wheels and Tires/VDBS/Tire2Veh/Wheel to Body Transform/Rotation Angles to Direction Cosine Matrix Retro: ZYX/Subsystem ==
  In1 : Inport
  In2 : Inport  Port=2
  In3 : Inport  Port=3
  In4 : Inport  Port=4
  In5 : Inport  Port=5
  In6 : Inport  Port=6
  In7 : Inport  Port=7
  In8 : Inport  Port=8
  In9 : Inport  Port=9
  Reshape : Reshape  OutputDimensionality=Customize  OutputDimensions=[3, 3]
  Vector Concatenate : Concatenate  NumInputs=9
  Out1 : Outport
  wires:
  Reshape/1 -> Out1/1
  Vector Concatenate/1 -> Reshape/1
  In1/1 -> Vector Concatenate/1
  In4/1 -> Vector Concatenate/2
  In7/1 -> Vector Concatenate/3
  In2/1 -> Vector Concatenate/4
  In5/1 -> Vector Concatenate/5
  In8/1 -> Vector Concatenate/6
  In3/1 -> Vector Concatenate/7
  In6/1 -> Vector Concatenate/8
  In9/1 -> Vector Concatenate/9

== system CAVE_MachE_Simulink_250904/Vehicle Under Test3/Vehicle/Vehicle Dynamics/Vehicle 14DOF/Wheels and Tires/VDBS/Veh2Tire/Wheel to Body Transform/Rotation Angles to Direction Cosine Matrix Retro: ZYX/Subsystem ==
  In1 : Inport
  In2 : Inport  Port=2
  In3 : Inport  Port=3
  In4 : Inport  Port=4
  In5 : Inport  Port=5
  In6 : Inport  Port=6
  In7 : Inport  Port=7
  In8 : Inport  Port=8
  In9 : Inport  Port=9
  Reshape : Reshape  OutputDimensionality=Customize  OutputDimensions=[3, 3]
  Vector Concatenate : Concatenate  NumInputs=9
  Out1 : Outport
  wires:
  Reshape/1 -> Out1/1
  Vector Concatenate/1 -> Reshape/1
  In1/1 -> Vector Concatenate/1
  In4/1 -> Vector Concatenate/2
  In7/1 -> Vector Concatenate/3
  In2/1 -> Vector Concatenate/4
  In5/1 -> Vector Concatenate/5
  In8/1 -> Vector Concatenate/6
  In3/1 -> Vector Concatenate/7
  In6/1 -> Vector Concatenate/8
  In9/1 -> Vector Concatenate/9

== system CAVE_MachE_Simulink_250904/Vehicle Under Test4/Vehicle/Vehicle Dynamics/Vehicle 14DOF/Wheels and Tires/VDBS/Tire2Veh/Wheel to Body Transform/Rotation Angles to Direction Cosine Matrix Retro: ZYX/Subsystem ==
  In1 : Inport
  In2 : Inport  Port=2
  In3 : Inport  Port=3
  In4 : Inport  Port=4
  In5 : Inport  Port=5
  In6 : Inport  Port=6
  In7 : Inport  Port=7
  In8 : Inport  Port=8
  In9 : Inport  Port=9
  Reshape : Reshape  OutputDimensionality=Customize  OutputDimensions=[3, 3]
  Vector Concatenate : Concatenate  NumInputs=9
  Out1 : Outport
  wires:
  In9/1 -> Vector Concatenate/9
  In6/1 -> Vector Concatenate/8
  In3/1 -> Vector Concatenate/7
  In8/1 -> Vector Concatenate/6
  In5/1 -> Vector Concatenate/5
  In2/1 -> Vector Concatenate/4
  In7/1 -> Vector Concatenate/3
  In4/1 -> Vector Concatenate/2
  In1/1 -> Vector Concatenate/1
  Vector Concatenate/1 -> Reshape/1
  Reshape/1 -> Out1/1

== system CAVE_MachE_Simulink_250904/Vehicle Under Test4/Vehicle/Vehicle Dynamics/Vehicle 14DOF/Wheels and Tires/VDBS/Veh2Tire/Wheel to Body Transform/Rotation Angles to Direction Cosine Matrix Retro: ZYX/Subsystem ==
  In1 : Inport
  In2 : Inport  Port=2
  In3 : Inport  Port=3
  In4 : Inport  Port=4
  In5 : Inport  Port=5
  In6 : Inport  Port=6
  In7 : Inport  Port=7
  In8 : Inport  Port=8
  In9 : Inport  Port=9
  Reshape : Reshape  OutputDimensionality=Customize  OutputDimensions=[3, 3]
  Vector Concatenate : Concatenate  NumInputs=9
  Out1 : Outport
  wires:
  In9/1 -> Vector Concatenate/9
  In6/1 -> Vector Concatenate/8
  In3/1 -> Vector Concatenate/7
  In8/1 -> Vector Concatenate/6
  In5/1 -> Vector Concatenate/5
  In2/1 -> Vector Concatenate/4
  In7/1 -> Vector Concatenate/3
  In4/1 -> Vector Concatenate/2
  In1/1 -> Vector Concatenate/1
  Vector Concatenate/1 -> Reshape/1
  Reshape/1 -> Out1/1

== matlab function CAVE_MachE_Simulink_250904/RealSim1/MATLAB Function3 ==
  data: simState input; connectionState input; timeSimulator input; timeStepSimulator output; timeStepSimulatorPrevious input; timeStepTrigger output
function [timeStepSimulator, timeStepTrigger]  = fcn(simState, connectionState, timeSimulator, timeStepSimulatorPrevious)


if simState && abs(connectionState-3) < 1e-5 && (timeSimulator >= timeStepSimulatorPrevious + 0.1 - 1e-5 || abs(timeSimulator) < 1e-5)
    timeStepSimulator = timeSimulator;
    timeStepTrigger = 1;
else
    timeStepSimulator = timeStepSimulatorPrevious;
    timeStepTrigger = 0;
end

== matlab function CAVE_MachE_Simulink_250904/RealSim1/MATLAB Function ==
  data: strUint8Vec input; intVal output double; strLen input
function intVal = strVec2Int(strUint8Vec, strLen)

    strVec = blanks(50);
    for i = 1:strLen
       strVec(i) = strUint8Vec(i); 
    end
    if strLen > 0
        intVal = real(str2double(strVec(1:strLen)));
    else
        intVal = -1;
    end

== matlab function CAVE_MachE_Simulink_250904/RealSim1/MATLAB Function1 ==
  data: strUint8Vec input; intVal output double; strLen input
function intVal = strVec2Int(strUint8Vec, strLen)

    strVec = blanks(50);
    for i = 1:strLen
       strVec(i) = strUint8Vec(i); 
    end
    if strLen > 0
        intVal = real(str2double(strVec(1:strLen)));
    else
        intVal = -1;
    end

== matlab function CAVE_MachE_Simulink_250904/RealSim1/MATLAB Function2 ==
  data: signalLightId input uint8 size=[1 50]; signalLightIdString output string; signalLightIdLength input
function signalLightIdString = fcn(signalLightId, signalLightIdLength)

signalLightIdString = string(char(signalLightId));

== matlab function CAVE_MachE_Simulink_250904/RealSim1/MATLAB Function4 ==
  data: simState input; simulatorStartTime output; simStatePrevious input; connectionState input; simulationTime input; simState output
function [simulatorStartTime, simState] = fcn(simState, simStatePrevious, connectionState, simulationTime)


if abs(simState - 1) < 1e-5 && abs(simStatePrevious) < 1e-5 && abs(connectionState-3) < 1e-5
    % set connectionState and start time
    simulatorStartTime = simulationTime;
else
    simulatorStartTime = 0;
end

== matlab function CAVE_MachE_Simulink_250904/RealSim2/MATLAB Function ==
  data: strUint8Vec input; intVal output double; strLen input
function intVal = strVec2Int(strUint8Vec, strLen)

    strVec = blanks(50);
    for i = 1:strLen
       strVec(i) = strUint8Vec(i); 
    end
    if strLen > 0
        intVal = real(str2double(strVec(1:strLen)));
    else
        intVal = -1;
    end

== matlab function CAVE_MachE_Simulink_250904/RealSim2/MATLAB Function1 ==
  data: strUint8Vec input; intVal output double; strLen input
function intVal = strVec2Int(strUint8Vec, strLen)

    strVec = blanks(50);
    for i = 1:strLen
       strVec(i) = strUint8Vec(i); 
    end
    if strLen > 0
        intVal = real(str2double(strVec(1:strLen)));
    else
        intVal = -1;
    end

== matlab function CAVE_MachE_Simulink_250904/RealSim2/MATLAB Function2 ==
  data: signalLightId input uint8 size=[1 50]; signalLightIdString output string; signalLightIdLength input
function signalLightIdString = fcn(signalLightId, signalLightIdLength)

signalLightIdString = string(char(signalLightId));

== matlab function CAVE_MachE_Simulink_250904/RealSim2/MATLAB Function3 ==
  data: simState input; connectionState input; timeSimulator input; timeStepSimulator output; timeStepSimulatorPrevious input; timeStepTrigger output
function [timeStepSimulator, timeStepTrigger]  = fcn(simState, connectionState, timeSimulator, timeStepSimulatorPrevious)


if simState && abs(connectionState-3) < 1e-5 && (timeSimulator >= timeStepSimulatorPrevious + 0.1 - 1e-5 || abs(timeSimulator) < 1e-5)
    timeStepSimulator = timeSimulator;
    timeStepTrigger = 1;
else
    timeStepSimulator = timeStepSimulatorPrevious;
    timeStepTrigger = 0;
end

== matlab function CAVE_MachE_Simulink_250904/RealSim2/MATLAB Function4 ==
  data: simState input; simulatorStartTime output; simStatePrevious input; connectionState input; simulationTime input; simState output
function [simulatorStartTime, simState] = fcn(simState, simStatePrevious, connectionState, simulationTime)


if abs(simState - 1) < 1e-5 && abs(simStatePrevious) < 1e-5 && abs(connectionState-3) < 1e-5
    % set connectionState and start time
    simulatorStartTime = simulationTime;
else
    simulatorStartTime = 0;
end

== stateflow chart CAVE_MachE_Simulink_250904/Vehicle Under Test1/Vehicle/Actuation and Outputs/MOOG Brake Actuator/MOOG Interface/MOOG State Machine ==
  state MainStateMachine [parallel]
    settings: executionOrder=2
    state Learning
      state LearnMinStop
        en:
        state BackStopCmd
          en:
          MoogOpMode=21 ;
          PositionCmd=-100000;
        state BackStopReached
          en:
          MoogOpMode=22;
          PositionCmd=0;
        state BackStopSettle
          en:
          MoogOpMode=23;
          MinStop=ActualPosition_cnt;
          PositionCmd=0;
        (default) -> MainStateMachine.Learning.LearnMinStop.BackStopCmd
        MainStateMachine.Learning.LearnMinStop.BackStopCmd -> MainStateMachine.Learning.LearnMinStop.BackStopReached : [bitand(StatusWord,8)]
        MainStateMachine.Learning.LearnMinStop.BackStopReached -> MainStateMachine.Learning.LearnMinStop.BackStopSettle : after(2,sec)
      state StartLearning
        en:
        MoogOpMode=11;
        PositionCmd=0;
        MinStop=-200000;
        MaxStop=200000;
      state LearnMaxStop
        en:
        state BackStopCmd
          en:
          MoogOpMode=31;
          PositionCmd=100000;
        state BackStopReached
          en:
          MoogOpMode=32;
          PositionCmd=0;
        state BackStopSettle
          en:
          MoogOpMode=33;
          MaxStop=ActualPosition_cnt;
          PositionCmd=0;
        (default) -> MainStateMachine.Learning.LearnMaxStop.BackStopCmd
        MainStateMachine.Learning.LearnMaxStop.BackStopCmd -> MainStateMachine.Learning.LearnMaxStop.BackStopReached : [bitand(StatusWord,8)]
        MainStateMachine.Learning.LearnMaxStop.BackStopReached -> MainStateMachine.Learning.LearnMaxStop.BackStopSettle : after(2,sec)
      state EndLearning
        en:
        MoogOpMode=41;
        PositionCmd=0;
        LearningComplete=1;
        FaultCntr=0;
      (default) -> StartLearning
      StartLearning -> LearnMinStop : after(0.5,sec)[InitComplete ==1]
      LearnMinStop -> LearnMaxStop : after(1,sec)[InitComplete ==1  && MinStop ~=-200000]
      LearnMaxStop -> EndLearning : after(1,sec)[InitComplete ==1  && MaxStop ~=200000 && ((MaxStop-MinStop)>ActuatorMinTravelForReady)]
    state NormalOperation
      state LearningNotComplete
        en:
        MoogOpMode=101;
        Actuator_Ready=0;
        du:
        PositionCmd=0;
      state LearningComplete
        en:
        MoogOpMode=102;
        Actuator_Ready=1;
        du:
        PositionCmd=TargetPosition_cnt;
      (default) -> LearningNotComplete
      LearningNotComplete -> LearningComplete : after(1,sec)[LearningComplete==1]
    MainStateMachine.Learning.LearnMaxStop.BackStopSettle -> NormalOperation : after(10,sec)
    Learning -> NormalOperation : after(1,sec)[LearningComplete==1]
    NormalOperation -> Learning : [PositionLearningTrigger==1]{Actuator_Ready =0;
        | LearningComplete=0}
    (default) -> NormalOperation : {Actuator_Ready =0;
        | LearningComplete=0}
  state MoogStateMachine [parallel]
    settings: executionOrder=1
    state Initialisation
      state SwitchOffDisabled
        % StatusWord= xxxx_xxxx_x0xx_0000, 0x00, 0d
        en:
        MoogSMState=13;
        ControlWord=0; % 0x00
      state Init
        en:
        MoogSMState=11;
        ControlWord=0;
        InitComplete =0;
      state ClearFault
        en:
        MoogSMState=12;
        ControlWord=128; % 0x80
      state SwitchOnDisabled
        % StatusWord= xxxx_xxxx_x1xx_0000, 0x40, 64d
        en:
        MoogSMState=14;
        ControlWord=6; % 0x06
      state ReadyToSwitchOn
        % StatusWord=xxxx_xxxx_x01x_0001, 0x21, 33d
        en:
        MoogSMState=15;
        ControlWord=7; % 0x07
      state SwitchedOn
        % StatusWord=xxxx_xxxx_x01x_0011, 0x23, 35d
        en:
        MoogSMState=16;
        ControlWord=15; % 0x0F
      state OperationEnabled
        % StatusWord=xxxx_xxxx_x01x_0111, 0x27, 39d
        en:
        MoogSMState=17;
        ControlWord=15; % 0x0F
        InitComplete=1;
      SwitchOffDisabled -> Init [order 2] : after(1,sec)[bitand(StatusWord,8)]{FaultCntr=FaultCntr+1;}
      (default) -> Init
      Init -> ClearFault : after(0.5,sec)
      ClearFault -> SwitchOffDisabled : after(0.5,sec)
      SwitchOffDisabled -> SwitchOnDisabled [order 1] : after(0.1,sec)[bitand(StatusWord,64)]
      OperationEnabled -> Init : after(1,sec)[bitand(StatusWord,8)]{FaultCntr=FaultCntr+1;}
      SwitchedOn -> Init [order 2] : after(1,sec)[bitand(StatusWord,8)]{FaultCntr=FaultCntr+1;}
      ReadyToSwitchOn -> Init [order 2] : after(1,sec)[bitand(StatusWord,8)]{FaultCntr=FaultCntr+1;}
      SwitchOnDisabled -> Init [order 2] : after(1,sec)[bitand(StatusWord,8)]{FaultCntr=FaultCntr+1;}
      SwitchOnDisabled -> ReadyToSwitchOn [order 1] : after(0.1,sec)[bitand(StatusWord,32) &...
          |  bitand(StatusWord,1)]
      ReadyToSwitchOn -> SwitchedOn [order 1] : after(0.1,sec)[bitand(StatusWord,32) & ...
          | bitand(StatusWord,2) & ...
          | bitand(StatusWord,1)]
      SwitchedOn -> OperationEnabled [order 1] : after(0.1,sec)[bitand(StatusWord,32) & ...
          | bitand(StatusWord,4) & ...
          | bitand(StatusWord,2) & ...
          | bitand(StatusWord,1)]
    state Wait
      en:
      MoogSMState=31;
      Actuator_Ready=0;
      InitComplete =0;
      LearningComplete=0;
    state PositionControl
      state EnableSetPoint
        en:
        MoogSMState=21;
        ControlWord=47; % 0x2F
      state BeginMotion
        en:
        MoogSMState=22;
        ControlWord=63; % 0x3F
      (default) -> EnableSetPoint
      EnableSetPoint -> BeginMotion : after(0.001,sec)[Actuator_Ready==1 || ...
          | MoogOpMode==21 || ...
          | MoogOpMode==31]
      BeginMotion -> EnableSetPoint : after(0.001,sec)
    Initialisation -> Wait [order 2] : after(2,sec)[CAN_CommsOK_Flg ==0]
    (default) -> Initialisation : {FaultCntr=0;}
    Initialisation -> Wait [order 3] : [FaultCntr>=5]
    Wait -> Initialisation : [ResetCmd &&CAN_CommsOK_Flg==1 ]{Actuator_Ready=0;FaultCntr=0;}
    Initialisation -> PositionControl [order 1] : [InitComplete==1]
    PositionControl -> Initialisation [order 1] : [ResetCmd ]{InitComplete=0;}
    PositionControl -> Initialisation [order 2] : [bitand(StatusWord,8)]{InitComplete=0;FaultCntr=FaultCntr+1;}
  data: CAN_CommsOK_Flg input; ControlWord output; PositionCmd output; ResetCmd input; PositionLearningTrigger input; StatusWord input; Actuator_Ready output; FaultCntr output; MoogSMState output; InitComplete output; MoogOpMode output; LearningComplete output; ActualPosition_cnt input; MaxStop output; MinStop output; TargetPosition_cnt input; ActuatorMinTravelForReady input

== matlab function CAVE_MachE_Simulink_250904/Vehicle Under Test1/Vehicle/Rototest and ORNL Interface/Get Wheel Spd Cmd Based on Wheel Dynamics/Whl Dynamics & Format CM Powertrain Signal/Subsystem/MATLAB Function ==
  data: axleTorq input; switchFlag output; wheelSpd input
function switchFlag = fcn(axleTorq, wheelSpd)

% if braking and vehicle has stopped
if (abs(axleTorq) < 1e-5 && abs(wheelSpd) < 1e-5)
    switchFlag = 1;
else
    switchFlag = 0;
end

== matlab function CAVE_MachE_Simulink_250904/Vehicle Under Test1/Vehicle/Rototest and ORNL Interface/Get Wheel Spd Cmd Based on Wheel Dynamics/Whl Dynamics & Format CM Powertrain Signal/Subsystem2/MATLAB Function ==
  data: axleTorq input; switchFlag output; wheelSpd input
function switchFlag = fcn(axleTorq, wheelSpd)

% if braking and vehicle has stopped
if (abs(axleTorq) < 1e-5 && abs(wheelSpd) < 1e-5)
    switchFlag = 1;
else
    switchFlag = 0;
end

== matlab function CAVE_MachE_Simulink_250904/Vehicle Under Test1/Vehicle/Rototest and ORNL Interface/Get Wheel Spd Cmd Based on Wheel Dynamics/Whl Dynamics & Format CM Powertrain Signal/Subsystem3/MATLAB Function ==
  data: axleTorq input; switchFlag output; wheelSpd input
function switchFlag = fcn(axleTorq, wheelSpd)

% if braking and vehicle has stopped
if (abs(axleTorq) < 1e-5 && abs(wheelSpd) < 1e-5)
    switchFlag = 1;
else
    switchFlag = 0;
end

== matlab function CAVE_MachE_Simulink_250904/Vehicle Under Test1/Vehicle/Rototest and ORNL Interface/Get Wheel Spd Cmd Based on Wheel Dynamics/Whl Dynamics & Format CM Powertrain Signal/Subsystem4/MATLAB Function ==
  data: axleTorq input; switchFlag output; wheelSpd input
function switchFlag = fcn(axleTorq, wheelSpd)

% if braking and vehicle has stopped
if (abs(axleTorq) < 1e-5 && abs(wheelSpd) < 1e-5)
    switchFlag = 1;
else
    switchFlag = 0;
end

== stateflow chart CAVE_MachE_Simulink_250904/Vehicle Under Test1/Vehicle/Rototest and ORNL Interface/To Rototest with Band-Aid/Band-Aid/Band-Aid ==
  state dStop
    en:
    OutMode = 0;
    State = 3;
  state Running
    state SpeedMode
      en:
      OutMode = 1;
      state Blend
        en:
        OutSpd = InSpd;
        State = 0.1;
      state Driving
        du:
        OutSpd = InSpd;
        State = 0.2;
      (default) -> Blend
      Blend -> Driving
    state TorqueMode
      en:
      OutMode = 0;
      du:
      State = 1;
    (default) -> SpeedMode
    TorqueMode -> Blend : [after(SettleTime, sec) || ...
        | ~BrkSw]
    SpeedMode -> TorqueMode : [(any(InSpd < SpdLatchThr) && ...
        | (VehSpd_kph < VehSpdThr_kph) && BrkSw)]
  note: The vehicle will enter speed mode (driving) if:
      | The vehicle has been in torque mode for a calibrated time (settleTime) AND
      | The Input Speed (InSpd) is greater than a Launch Treshold (LaunchSpdThr) OR
      | The Input Torque (InTrq) is greater than calibrated torque value (LaunchTrqThr).
      | Criteria 1) sees the dyno has "settled" and allows the dyno to go back into speed mode.
      | Criteria 2) sees the vehicle is attempting to reaccelerate and pushes into speed mode.
      |
      | The vehicle will enter torque mode (zero) if:
      | Input Speed (InSpd) goes below the calibrated speed (SpdLatchThr) AND
      | Brake (BrkSw) is active.
      | 2) dStop is activated.
      | Criteria 1) sees the vehicle is attempting to come to a stop and unloads the dyno.
      | Criteria 2) is SHTF.
      |
      | && ...
      | (InSpd > LaunchSpdThr || ...
      | InTrq > LaunchTrqThr)
  (default) -> dStop
  Running -> dStop : [dStop]
  dStop -> Running : [~dStop]
  data: LaunchSpdThr input; LaunchTrqThr input; SpdLatchThr input; BrkSw input; InSpd input; InTrq input; OutMode output size=1; OutSpd output; State output; SettleTime input; dStop input; VehSpd_kph input; VehSpdThr_kph input

== matlab function CAVE_MachE_Simulink_250904/Vehicle Under Test1/Vehicle/Rototest and ORNL Interface/To Rototest with Band-Aid/RotoTestEthTx/MATLAB Function ==
  data: SpTqRR input; y output; SpTqLR input; SpTqRF input; SpTqLF input; SystemActive input
function y = fcn(SpTqRR, SpTqLR, SpTqRF, SpTqLF, SystemActive)

y = 0;
if SpTqRR == 1 && SystemActive == 0
    y = 30;
elseif SpTqRR == 0 && SystemActive == 0
    y = 0;
elseif SpTqRR == 1 && SystemActive == 1
    y = 31;
elseif SpTqRR == 0 && SystemActive == 1
    y = 1;
end

y = uint8(y);

== matlab function CAVE_MachE_Simulink_250904/Vehicle Under Test1/Vehicle/Vehicle Dynamics/Vehicle 14DOF/Wheels and Tires/VDBS/Tires/MF Tires/MATLAB Function ==
  data: axleTorq input; switchFlag output; wheelSpd input
function switchFlag = fcn(axleTorq, wheelSpd)

% if braking and vehicle has stopped
%if (abs(axleTorq) < 1e-5 && abs(wheelSpd) < 1e-5)
if abs(wheelSpd) < 1e-5
    switchFlag = 1;
else
    switchFlag = 0;
end
